simulink model "untitled"  (R2016b)
settings: Solver=FixedStepAuto  StartTime=0.0  StopTime=10.0  FixedStep=0.0005  RelTol=1e-3
settings Model: Creator=Ross Hartley  LastModifiedBy=Ross Hartley

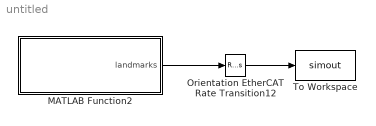
== system untitled ==
  MATLAB Function2 : MATLAB Function  TreatAsAtomicUnit=on
  Orientation EtherCAT Rate Transition12 : RateTransition  Deterministic=off  OutPortSampleTime=1/1000
  To Workspace : ToWorkspace  VariableName=simout  SaveFormat=Structure With Time  SampleTime=-1
  wires:
  MATLAB Function2/1(landmarks) -> Orientation EtherCAT Rate Transition12/1
  Orientation EtherCAT Rate Transition12/1 -> To Workspace/1

== matlab function untitled/MATLAB Function2 ==
  settings: updateMethod=DISCRETE  sampleTime=1/2000
  data: landmarks output size=[4,10]
function landmarks = SpoofNoLandmarks()

% Initialize landmarks
landmarks = nan(4,10);
landmarks(:,1) = [0;0;0;1];
% landmarks = [0;0;0;1];

end
